simulink model "PlantModel"  (R2022b)
settings: configuration reference "simConfigSet" (kept outside this file)
undefined symbols (not defined in the file): Earth, env, F, GPSTimeSeed, Light, MIL, sensors, uavData, WGS84
libraries: mbdriLib x22, aerolibactuator x5, aerolibasang x2, aerolibatmos2 x2, aerolibconvert2 x2, aerolibwind2 x2, shared6dof x1, aerolibnav x1, simulink x1, aerolibtransform2 x1
(part 1 of 2)
settings Model: Creator=promero  LastModifiedBy=nitinmiyyapuram
settings ConfigSetRef: SourceName=simConfigSet  SourceLocation=Base Workspace

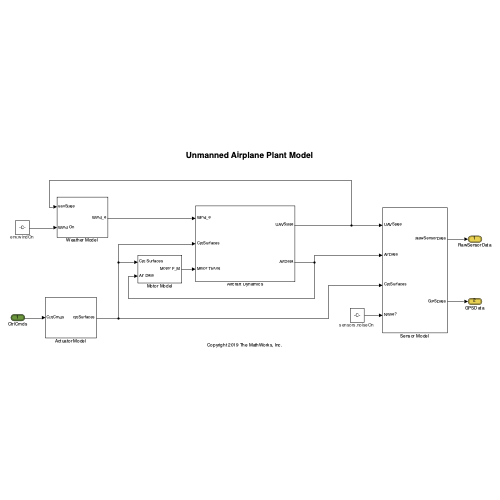
[thumbnail: Simulink's stored preview of the top-level diagram]
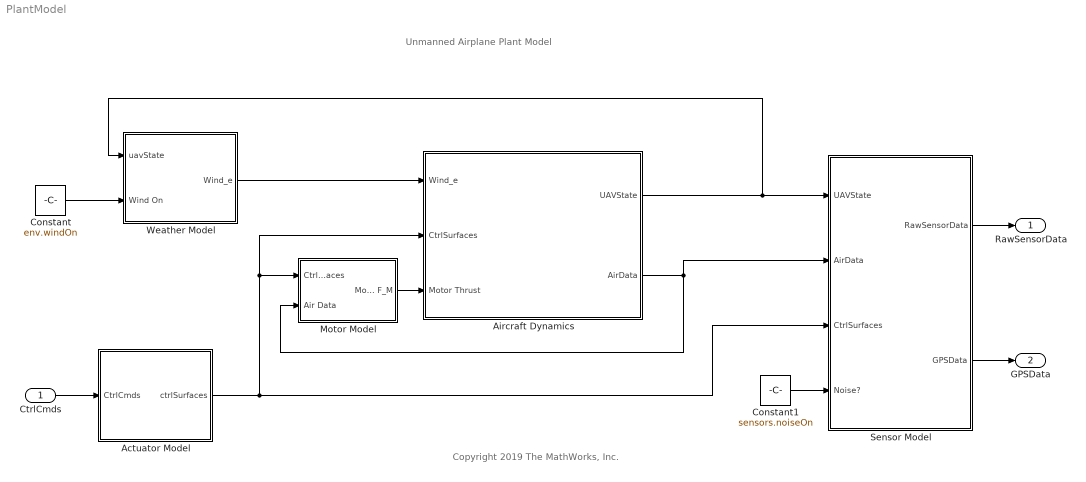
== system PlantModel ==
  note: Unmanned Airplane Plant Model
  note: Copyright 2019 The MathWorks, Inc.
  CtrlCmds : Inport  OutDataTypeStr=Bus: ctrlCmdsBus
  Actuator Model : Subsystem
  Aircraft Dynamics : Subsystem
  Constant : Constant  Value=env.windOn
      settings: AttributesFormatString=%<Value>
  Constant1 : Constant  Value=sensors.noiseOn
      settings: AttributesFormatString=%<Value>
  Motor Model : Subsystem
  Sensor Model : Subsystem
  Weather Model : Subsystem
  RawSensorData : Outport  OutDataTypeStr=Bus: rawSensorDataBus  PortDimensions=1  SampleTime=0  VectorParamsAs1DForOutWhenUnconnected=off  BusOutputAsStruct=on
  GPSData : Outport  Port=2  OutDataTypeStr=Bus: gpsReading  PortDimensions=1  VectorParamsAs1DForOutWhenUnconnected=off  BusOutputAsStruct=on
  wires:
  Sensor Model/2(GPSData) -> GPSData/1
  Weather Model/1(Wind_e) -> Aircraft Dynamics/1(Wind_e)
  Sensor Model/1(RawSensorData) -> RawSensorData/1
  Constant1/1 -> Sensor Model/4(Noise?)
  Constant/1 -> Weather Model/2(Wind On)
  Aircraft Dynamics/1(UAVState) -> Weather Model/1(uavState), Sensor Model/1(UAVState)
  CtrlCmds/1 -> Actuator Model/1(CtrlCmds)
  Actuator Model/1(ctrlSurfaces) -> Sensor Model/3(CtrlSurfaces), Aircraft Dynamics/2(CtrlSurfaces), Motor Model/1(Ctrl Surfaces)
  Motor Model/1(Motor F_M) -> Aircraft Dynamics/3(Motor Thrust)
  Aircraft Dynamics/2(AirData) -> Motor Model/2(Air Data), Sensor Model/2(AirData)

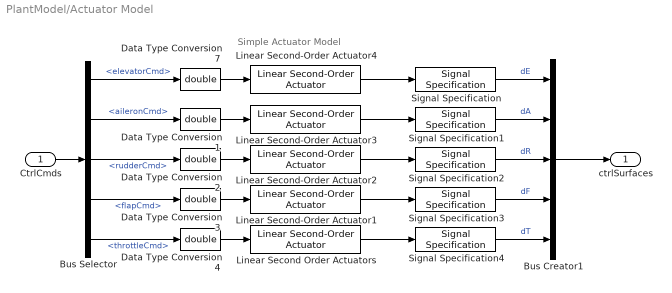
== system PlantModel/Actuator Model ==
  note: Simple Actuator Model
  CtrlCmds : Inport
  Bus Creator1 : BusCreator  Inputs=5
  Bus Selector : BusSelector  OutputSignals=elevatorCmd,aileronCmd,rudderCmd,flapCmd,throttleCmd
  Data Type Conversion{1..4,7} (5 alike) : DataTypeConversion  OutDataTypeStr=double  SaturateOnIntegerOverflow=off  RndMeth=Floor
  Linear Second Order Actuators : aerolibactuator/Linear Second-Order Actuator  wn_fin=35  z_fin=0.75  fin_act_0=0  fin_act_vel=0
      settings: AttributesFormatString=|
      | Nat Freq => %<wn_fin>
      | Damping => %<z_fin>
  Linear Second-Order Actuator{1..4} (4 alike) : aerolibactuator/Linear Second-Order Actuator  wn_fin=35  z_fin=0.75  fin_act_0=0  fin_act_vel=0
  Signal Specification{,1..3} (4 alike) : SignalSpecification  Unit=rad
  Signal Specification4 : SignalSpecification  Unit=%
  ctrlSurfaces : Outport  VectorParamsAs1DForOutWhenUnconnected=off
  wires:
  CtrlCmds/1 -> Bus Selector/1
  Data Type Conversion7/1 -> Linear Second-Order Actuator4/1
  Data Type Conversion1/1 -> Linear Second-Order Actuator3/1
  Data Type Conversion2/1 -> Linear Second-Order Actuator2/1
  Data Type Conversion3/1 -> Linear Second-Order Actuator1/1
  Data Type Conversion4/1 -> Linear Second Order Actuators/1
  Bus Creator1/1 -> ctrlSurfaces/1
  Bus Selector/1 -> Data Type Conversion7/1  "<elevatorCmd>"
  Linear Second-Order Actuator2/1 -> Signal Specification2/1
  Linear Second-Order Actuator3/1 -> Signal Specification1/1
  Linear Second-Order Actuator1/1 -> Signal Specification3/1
  Linear Second-Order Actuator4/1 -> Signal Specification/1
  Bus Selector/4 -> Data Type Conversion3/1  "<flapCmd>"
  Bus Selector/5 -> Data Type Conversion4/1  "<throttleCmd>"
  Bus Selector/3 -> Data Type Conversion2/1  "<rudderCmd>"
  Bus Selector/2 -> Data Type Conversion1/1  "<aileronCmd>"
  Linear Second Order Actuators/1 -> Signal Specification4/1
  Signal Specification/1 -> Bus Creator1/1  "dE"
  Signal Specification1/1 -> Bus Creator1/2  "dA"
  Signal Specification2/1 -> Bus Creator1/3  "dR"
  Signal Specification3/1 -> Bus Creator1/4  "dF"
  Signal Specification4/1 -> Bus Creator1/5  "dT"

== system PlantModel/Aircraft Dynamics ==
  Wind_e : Inport
  CtrlSurfaces : Inport  Port=2
  Motor Thrust : Inport  Port=3
  6DOF Equations of Motion : Subsystem  VariantControl=use_aerospace_blocks == 1
  Aerodynamic Forces and Moments : Subsystem
  Sum : Sum  Inputs=++|  SaturateOnIntegerOverflow=on
  UAVState : Outport  VectorParamsAs1DForOutWhenUnconnected=off
  AirData : Outport  Port=2  VectorParamsAs1DForOutWhenUnconnected=off
  wires:
  Aerodynamic Forces and Moments/1(AirData) -> AirData/1
  6DOF Equations of Motion/1(UAVState) -> UAVState/1, Aerodynamic Forces and Moments/3(UAVState)
  Aerodynamic Forces and Moments/2(FM_b) -> Sum/2
  Sum/1 -> 6DOF Equations of Motion/1(FM_b)
  CtrlSurfaces/1 -> Aerodynamic Forces and Moments/1(CtrlSurfaces)
  Wind_e/1 -> Aerodynamic Forces and Moments/2(Wind_e)
  Motor Thrust/1 -> Sum/1

== system PlantModel/Motor Model ==
  Ctrl Surfaces : Inport
  Air Data : Inport  Port=2
  Bus Selector : BusSelector  OutputSignals=dT
  Bus Selector1 : BusSelector  OutputSignals=airpseed
  Constant : Constant  Value=[0 0 0]
  Engine Model : Subsystem
  Mux : Mux  Inputs=2
  Motor F_M : Outport  VectorParamsAs1DForOutWhenUnconnected=off
  wires:
  Bus Selector1/1 -> Engine Model/2(Airspeed)  "<airpseed>"
  Ctrl Surfaces/1 -> Bus Selector/1
  Engine Model/1(Thrust_b) -> Mux/1
  Constant/1 -> Mux/2
  Air Data/1 -> Bus Selector1/1
  Bus Selector/1 -> Engine Model/1(dt)  "<dT>"
  Mux/1 -> Motor F_M/1

== system PlantModel/Sensor Model ==
  UAVState : Inport
  AirData : Inport  Port=2
  CtrlSurfaces : Inport  Port=3
  Noise? : Inport  Port=4  OutDataTypeStr=double  PortDimensions=1
  "Air Sensor Model " : Subsystem
  Assemble GPS and State Data : Subsystem
  Noise Model : Subsystem  TreatAsAtomicUnit=on
  Sampling Model : Subsystem  TreatAsAtomicUnit=on
  RawSensorData : Outport  OutDataTypeStr=Bus: rawSensorDataBus  PortDimensions=1  SampleTime=0  VectorParamsAs1DForOutWhenUnconnected=off  BusOutputAsStruct=on
  GPSData : Outport  Port=2  OutDataTypeStr=Bus: gpsReading  PortDimensions=1  VectorParamsAs1DForOutWhenUnconnected=off  BusOutputAsStruct=on
  wires:
  Sampling Model/2(GPSData) -> GPSData/1
  Sampling Model/1(RawSensorData) -> RawSensorData/1
  CtrlSurfaces/1 -> Assemble GPS and State Data/3(CtrlSurfaces)
  UAVState/1 -> Assemble GPS and State Data/1(UAVState), "Air Sensor Model "/1(uavState)
  Assemble GPS and State Data/1(UAVStateBus) -> Noise Model/1(UAVState)  "uavState"
  Noise?/1 -> Noise Model/2(Noise?)
  Noise Model/1(SensorData) -> Sampling Model/1(Sensor Data)
  AirData/1 -> "Air Sensor Model "/2(AirData)
  "Air Sensor Model "/1(AirSensorData) -> Assemble GPS and State Data/2(AirSensorData)

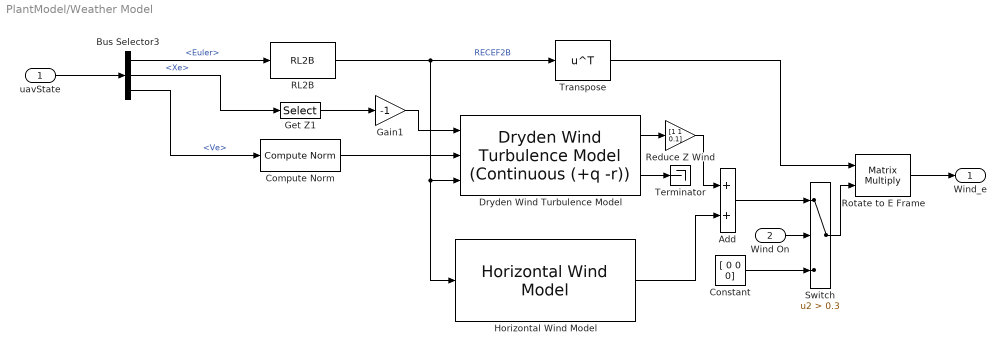
== system PlantModel/Weather Model ==
  uavState : Inport
  Wind On : Inport  Port=2
  " Compute Norm" : mbdriLib/Utilities/ Compute Norm  SystemSampleTime=-1  VariantActivationTime=update diagram  Latency=0  AutoFrameSizeCalculation=off
  Add : Sum  Inputs=2
  Bus Selector3 : BusSelector  OutputSignals=Euler,Xe,Ve
  Constant : Constant  Value=[ 0 0 0]
      settings: AttributesFormatString=%<Value>
  Dryden Wind Turbulence Model : aerolibwind2/Dryden Wind Turbulence Model  (Continuous (+q -r))  units=Metric (MKS)  spec=MIL-F-8785C  model=Continuous Dryden (+q -r)  W20=env.windBase/4  Wdeg=env.windDirTurb  TurbProb=10^-2 - Light  L_high=533.4  Wingspan=uavData.geometry.span  ts=ap.apSampleTime  Seed=[23341 23342 23343 23344]  T_on=on
  Gain1 : Gain  Gain=-1
      settings: AttributesFormatString=Z to Alt
  Get Z1 : Selector  InputPortWidth=3  IndexOptions=Index vector (dialog)  Indices=[3]  OutputSizes=[(-2)]
  "Horizontal Wind Model " : aerolibwind2/Horizontal Wind Model  units=Metric (MKS)  Vw_source=Internal  Vwind=env.windBase  W_source=Internal  Wdeg=env.windDirHor
  RL2B : mbdriLib/Coordinates/RL2B  SystemSampleTime=-1  VariantActivationTime=update diagram  Latency=0  AutoFrameSizeCalculation=off
  Reduce Z Wind : Gain  Gain=[1 1 0.1]
      settings: AttributesFormatString=%<Gain>
  Rotate to E Frame : Product  Multiplication=Matrix(*)
  Switch : Switch  Criteria=u2 > Threshold  Threshold=0.3  SaturateOnIntegerOverflow=off  InputSameDT=off
  Terminator : Terminator
  Transpose : Math  Operator=transpose  SignedPower=on
  Wind_e : Outport  Unit=m/s  VectorParamsAs1DForOutWhenUnconnected=off
  wires:
  Bus Selector3/2 -> Get Z1/1  "<Xe>"
  Bus Selector3/1 -> RL2B/1  "<Euler>"
  Dryden Wind Turbulence Model/2 -> Terminator/1
  Constant/1 -> Switch/3
  Get Z1/1 -> Gain1/1
  Bus Selector3/3 -> " Compute Norm"/1  "<Ve>"
  RL2B/1 -> Dryden Wind Turbulence Model/3, "Horizontal Wind Model "/1, Transpose/1  "RECEF2B"
  Transpose/1 -> Rotate to E Frame/1
  Rotate to E Frame/1 -> Wind_e/1
  Switch/1 -> Rotate to E Frame/2
  Dryden Wind Turbulence Model/1 -> Reduce Z Wind/1
  " Compute Norm"/1 -> Dryden Wind Turbulence Model/2
  uavState/1 -> Bus Selector3/1
  Gain1/1 -> Dryden Wind Turbulence Model/1
  "Horizontal Wind Model "/1 -> Add/2
  Reduce Z Wind/1 -> Add/1
  Add/1 -> Switch/1
  Wind On/1 -> Switch/2

== system PlantModel/Aircraft Dynamics/6DOF Equations of Motion ==
  FM_b : Inport
  6DOF (Euler Angles) : shared6dof/6DOF (Euler Angles)  units=Metric (MKS)  mtype=Fixed  rep=Euler Angles  xme_0=uavData.ic.Pos_0.*[1; 1; -1]  Vm_0=uavData.ic.Vb_0  eul_0=uavData.ic.Euler_0  pm_0=uavData.ic.PQR_0  mass_0=uavData.geometry.mass  mass_e=0.5  mass_f=2.0  inertia=eye(3).*[uavData.inertia.Ixx;uavData.inertia.Iyy; uavData.inertia.Izz]  inertia_e=eye(3)  inertia_f=2*eye(3)  k_quat=1.0  vre_flag=on  abi_flag=off  aMode=aMode  xme_statename=''  Vm_statename=''  eul_statename=''  quat_statename=''  pm_statename=''  mass_statename=''
  Bus Creator : BusCreator  Inputs=7
  Compute psi_dot : Subsystem
  Constant : Constant  Value=[0 0 0]
      settings: AttributesFormatString=%<Value>
  Demux2 : Demux  Outputs=2
  Terminator1 : Terminator
  Three-axis Accelerometer : aerolibnav/Three-axis Accelerometer  units=Metric (MKS)  acc=[0 0 0]  gtype=off  dtype_a=off  w_a=190  z_a=0.707  a_sf_cc=[1 0 0; 0 1 0; 0 0 1]  a_bias=[0 0 0]  a_Ts=0  a_rand=off  a_seeds=[23093 23094 23095]  a_pow=[0.001 0.001 0.001]  a_sat="[-inf  -inf  -inf  inf inf inf]"
  "[0, pi] Wrap Around" : Subsystem
  UAVState : Outport  VectorParamsAs1DForOutWhenUnconnected=off
  wires:
  Three-axis Accelerometer/1 -> Bus Creator/6  "Ab"
  Constant/1 -> Three-axis Accelerometer/4
  "[0, pi] Wrap Around"/1(Wrapped) -> Bus Creator/3  "Euler"
  6DOF (Euler Angles)/8 -> Three-axis Accelerometer/1
  6DOF (Euler Angles)/5 -> Bus Creator/4  "Vb"
  6DOF (Euler Angles)/2 -> Bus Creator/2  "Xe"
  6DOF (Euler Angles)/1 -> Bus Creator/1  "Ve"
  Bus Creator/1 -> UAVState/1
  6DOF (Euler Angles)/7 -> Three-axis Accelerometer/3
  6DOF (Euler Angles)/4 -> Terminator1/1
  6DOF (Euler Angles)/3 -> Compute psi_dot/1(Euler), "[0, pi] Wrap Around"/1(Euler)
  6DOF (Euler Angles)/6 -> Compute psi_dot/2(G), Bus Creator/5, Three-axis Accelerometer/2  "pqr"
  FM_b/1 -> Demux2/1
  Demux2/2 -> 6DOF (Euler Angles)/2
  Demux2/1 -> 6DOF (Euler Angles)/1
  Compute psi_dot/1(psi_dot) -> Bus Creator/7  "psi_dot"

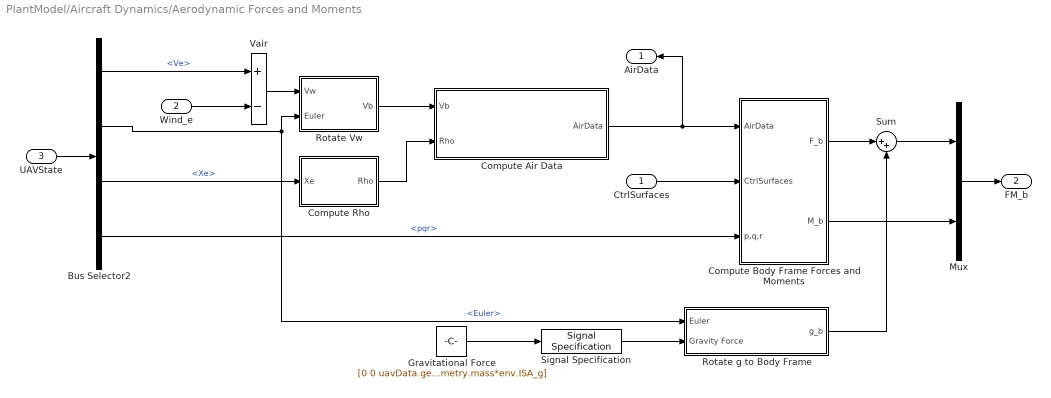
== system PlantModel/Aircraft Dynamics/Aerodynamic Forces and Moments ==
  CtrlSurfaces : Inport
  Wind_e : Inport  Port=2
  UAVState : Inport  Port=3
  Bus Selector2 : BusSelector  OutputSignals=Ve,Euler,Xe,pqr
  Compute Air Data : Subsystem  TreatAsAtomicUnit=on  VariantControl=use_aerospace_blocks == 1
  Compute Body Frame Forces and Moments : Subsystem
  Compute Rho : Subsystem
  Gravitational Force : Constant  Value=[0 0 uavData.geometry.mass*env.ISA_g]  VectorParams1D=off
      settings: AttributesFormatString=%<Value>
  Mux : Mux  Inputs=2
  Rotate Vw : Subsystem
  Rotate g to Body Frame : Subsystem
  Signal Specification : SignalSpecification  Unit=kg*m/s^2
  Sum : Sum  Inputs=|++  SaturateOnIntegerOverflow=on
  Vair : Sum  Inputs=+-  InputSameDT=on  SaturateOnIntegerOverflow=on  OutDataTypeStr=Inherit: Same as first input
  AirData : Outport  VectorParamsAs1DForOutWhenUnconnected=off
  FM_b : Outport  Port=2  VectorParamsAs1DForOutWhenUnconnected=off
  wires:
  Bus Selector2/1 -> Vair/1  "<Ve>"
  UAVState/1 -> Bus Selector2/1
  Mux/1 -> FM_b/1
  Sum/1 -> Mux/1
  Compute Body Frame Forces and Moments/1(F_b) -> Sum/1
  Rotate g to Body Frame/1(g_b) -> Sum/2
  Wind_e/1 -> Vair/2
  CtrlSurfaces/1 -> Compute Body Frame Forces and Moments/2(CtrlSurfaces)
  Compute Air Data/1(AirData) -> AirData/1, Compute Body Frame Forces and Moments/1(AirData)
  Bus Selector2/4 -> Compute Body Frame Forces and Moments/3(p,q,r)  "<pqr>"
  Gravitational Force/1 -> Signal Specification/1
  Compute Body Frame Forces and Moments/2(M_b) -> Mux/2
  Rotate Vw/1(Vb) -> Compute Air Data/1(Vb)
  Compute Rho/1(Rho) -> Compute Air Data/2(Rho)
  Bus Selector2/2 -> Rotate Vw/2(Euler), Rotate g to Body Frame/1(Euler)  "<Euler>"
  Vair/1 -> Rotate Vw/1(Vw)
  Signal Specification/1 -> Rotate g to Body Frame/2(Gravity Force)
  Bus Selector2/3 -> Compute Rho/1(Xe)  "<Xe>"

== system PlantModel/Motor Model/Engine Model ==
  dt : Inport
  Airspeed : Inport  Port=2
  Constant4 : Constant  Value=0
      settings: AttributesFormatString=%<Value>
  Get To : Subsystem
  Mass Conversion : aerolibconvert2/Mass Conversion  IU=lbm  OU=kg
  Mux : Mux  Inputs=2
  Mux1 : Mux  Inputs=3
  Thrust Available (lbs) : Fcn  Expr=u(1) - 0.047*sqrt(u(1))*u(2)
  kg2N : Gain  Gain=env.ISA_g  SaturateOnIntegerOverflow=on  OutDataTypeStr=Inherit: Same as input  ParamDataTypeStr=Inherit: Same as input
      settings: AttributesFormatString=%<Gain>
  Thrust_b : Outport  Unit=kg*m/s^2  VectorParamsAs1DForOutWhenUnconnected=off
  wires:
  kg2N/1 -> Mux1/1
  Constant4/1 -> Mux1/3, Mux1/2
  Mass Conversion/1 -> kg2N/1
  Mux1/1 -> Thrust_b/1
  Airspeed/1 -> Mux/2
  Thrust Available (lbs)/1 -> Mass Conversion/1
  Mux/1 -> Thrust Available (lbs)/1
  Get To/1(To) -> Mux/1
  dt/1 -> Get To/1(dt)

== system PlantModel/Sensor Model/Air Sensor Model  ==
  uavState : Inport
  AirData : Inport  Port=2
  Bus Creator : BusCreator  Inputs=4
  Bus Selector1 : BusSelector  OutputSignals=airpseed,q
  Bus Selector3 : BusSelector  OutputSignals=Xe
  Gain : Gain  Gain=-1
      settings: AttributesFormatString=Z to Alt
  Get Z : Selector  InputPortWidth=3  IndexOptions=Index vector (dialog)  Indices=[3]  OutputSizes=[(-2)]
  ISA Atmosphere Model1 : aerolibatmos2/ISA Atmosphere Model  custom=on  g=env.ISA_g  gamma=1.4  R=env.ISA_R  L=env.ISA_lapse  h_trop=11000  h_strat=20000  rho0=env.ISA_rho0  P0=env.ISA_P0  T0=env.ISA_T0  h0=0
  Terminator : Terminator
  Terminator1 : Terminator
  Transfer Fcn : TransferFcn  Denominator=[.01 1]
  Unit Conversion : UnitConversion  OutputType=Inherit: Inherit via back propagation
  AirSensorData : Outport  VectorParamsAs1DForOutWhenUnconnected=off
  wires:
  Bus Selector3/1 -> Get Z/1  "<Xe>"
  Get Z/1 -> Transfer Fcn/1
  Unit Conversion/1 -> Bus Creator/1  "OAT"
  Bus Selector1/1 -> Bus Creator/3  "<airpseed>"
  Bus Selector1/2 -> Bus Creator/4  "<q>"
  ISA Atmosphere Model1/1 -> Unit Conversion/1  "OAT"
  Bus Creator/1 -> AirSensorData/1
  Gain/1 -> ISA Atmosphere Model1/1
  ISA Atmosphere Model1/3 -> Bus Creator/2  "static"
  ISA Atmosphere Model1/2 -> Terminator1/1
  AirData/1 -> Bus Selector1/1
  Transfer Fcn/1 -> Gain/1
  uavState/1 -> Bus Selector3/1
  ISA Atmosphere Model1/4 -> Terminator/1

== system PlantModel/Sensor Model/Assemble GPS and State Data ==
  UAVState : Inport
  AirSensorData : Inport  Port=2
  CtrlSurfaces : Inport  Port=3
  Bus Creator : BusCreator  Inputs=11  OutDataTypeStr=Bus: uavStateBus  NonVirtualBus=on
      settings: InheritFromInputs=off
  Bus Creator1 : BusCreator  Inputs=5  OutDataTypeStr=Bus: gpsReading
      settings: InheritFromInputs=off
  Bus Selector : BusSelector  OutputSignals=static,q,OAT,airpseed
  Bus Selector1 : BusSelector  OutputSignals=dE,dA,dR,dF,dT
  Bus Selector2 : BusSelector  OutputSignals=Euler,pqr,Xe,Ve,Ab
  Bus Selector3 : BusSelector  OutputSignals=Xe,Ve
  Bus Selector4 : BusSelector  OutputSignals=gps_latLon,gps_h,gps_cog,gps_sog,gps_fix
  Generate GPS Data : Subsystem
  Mux : Mux  Inputs=5
  UAVStateBus : Outport  OutDataTypeStr=Bus: uavStateBus  VectorParamsAs1DForOutWhenUnconnected=off
  wires:
  Bus Creator1/1 -> Bus Creator/10
  Mux/1 -> Bus Creator/11  "ctrlSurfacePos"
  CtrlSurfaces/1 -> Bus Selector1/1  "ctrlSurfacePos"
  Bus Selector1/4 -> Mux/4  "<dF>"
  Bus Selector1/2 -> Mux/2  "<dA>"
  Bus Selector/4 -> Bus Creator/9  "<airpseed>"
  Bus Selector/2 -> Bus Creator/7  "<q>"
  Bus Selector/3 -> Bus Creator/8  "<OAT>"
  Bus Selector1/1 -> Mux/1  "<dE>"
  Bus Selector1/3 -> Mux/3  "<dR>"
  Bus Selector1/5 -> Mux/5  "<dT>"
  Bus Selector/1 -> Bus Creator/6  "<static>"
  Bus Creator/1 -> UAVStateBus/1
  AirSensorData/1 -> Bus Selector/1
  Bus Selector2/5 -> Bus Creator/5  "<Ab>"
  Bus Selector2/1 -> Bus Creator/1  "<Euler>"
  Bus Selector2/3 -> Bus Creator/3  "<Xe>"
  Bus Selector2/4 -> Bus Creator/4  "<Ve>"
  Bus Selector2/2 -> Bus Creator/2  "<pqr>"
  Bus Selector3/1 -> Generate GPS Data/1(XYZ (NEU))  "<Xe>"
  Bus Selector3/2 -> Generate GPS Data/2("Vx, Vy, Vz")  "<Ve>"
  Bus Selector4/5 -> Bus Creator1/5  "<gps_fix>"
  Bus Selector4/1 -> Bus Creator1/1  "<gps_latLon>"
  Bus Selector4/3 -> Bus Creator1/3  "<gps_cog>"
  Generate GPS Data/1(GPSData) -> Bus Selector4/1
  Bus Selector4/4 -> Bus Creator1/4  "<gps_sog>"
  Bus Selector4/2 -> Bus Creator1/2  "<gps_h>"
  UAVState/1 -> Bus Selector3/1, Bus Selector2/1

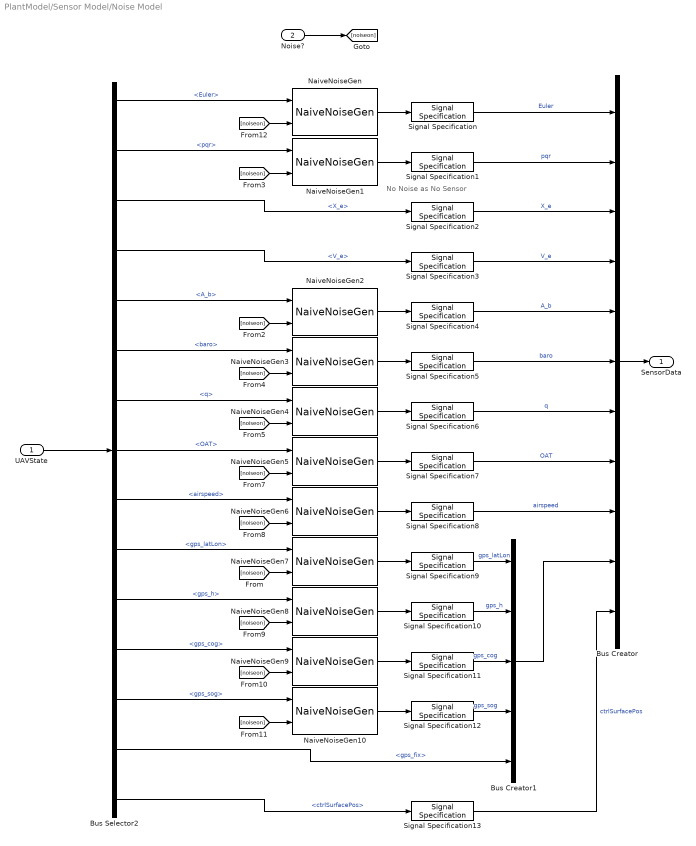
== system PlantModel/Sensor Model/Noise Model ==
  note: No Noise as No Sensor
  UAVState : Inport  OutDataTypeStr=Bus: uavStateBus
  Noise? : Inport  Port=2
  Bus Creator : BusCreator  Inputs=11  OutDataTypeStr=Bus: uavStateBus
      settings: InheritFromInputs=off
  Bus Creator1 : BusCreator  Inputs=5  OutDataTypeStr=Bus: gpsReading
      settings: InheritFromInputs=off
  Bus Selector2 : BusSelector  OutputSignals=Euler,pqr,X_e,V_e,A_b,baro,q,OAT,airspeed,gpsState.gps_latLon,gpsState.gps_h,gpsState.gps_cog,gpsState.gps_sog,gpsState.gps_fix,ctrlSurfacePos
  NaiveNoiseGen : mbdriLib/Utilities/NaiveNoiseGen  np=[0.0005 0.0005 0.0005]  st=ap.apSampleTime  ng=0.05  ns=[132 456 789]
  NaiveNoiseGen1 : mbdriLib/Utilities/NaiveNoiseGen  np=[0.0005 0.0005 0.0005]  st=ap.apSampleTime  ng=0.01  ns=[4132 4456 4789]
  NaiveNoiseGen10 : mbdriLib/Utilities/NaiveNoiseGen  np=[0.0005]  st=ap.apSampleTime  ng=0.1  ns=[8721]
  NaiveNoiseGen2 : mbdriLib/Utilities/NaiveNoiseGen  np=[0.0005 0.0005 0.0005]  st=ap.apSampleTime  ng=0.01  ns=[138 458 788]
  NaiveNoiseGen3 : mbdriLib/Utilities/NaiveNoiseGen  np=[0.0005]  st=ap.apSampleTime  ng=0.2  ns=[1387]
  NaiveNoiseGen4 : mbdriLib/Utilities/NaiveNoiseGen  np=[0.0005]  st=ap.apSampleTime  ng=0.15  ns=[1317]
  NaiveNoiseGen5 : mbdriLib/Utilities/NaiveNoiseGen  np=[0.0005]  st=ap.apSampleTime  ng=0.2  ns=[1917]
  NaiveNoiseGen6 : mbdriLib/Utilities/NaiveNoiseGen  np=[0.0005]  st=ap.apSampleTime  ng=0.15  ns=[1557]
  NaiveNoiseGen7 : mbdriLib/Utilities/NaiveNoiseGen  np=[0.0001 0.0001]  st=ap.apSampleTime  ng=0.00001  ns=[138 458]
  NaiveNoiseGen8 : mbdriLib/Utilities/NaiveNoiseGen  np=[0.0005]  st=ap.apSampleTime  ng=0.15  ns=[7757]
  NaiveNoiseGen9 : mbdriLib/Utilities/NaiveNoiseGen  np=[0.0005]  st=ap.apSampleTime  ng=0.15  ns=[8757]
  Signal Specification : SignalSpecification  Unit=rad
  Signal Specification1 : SignalSpecification  Unit=rad/s
  Signal Specification10 : SignalSpecification  Unit=m
  Signal Specification11 : SignalSpecification  Unit=deg
  Signal Specification12 : SignalSpecification  Unit=m/s
  Signal Specification13 : SignalSpecification  Unit=rad
  Signal Specification2 : SignalSpecification  Unit=m
  Signal Specification3 : SignalSpecification  Unit=m/s
  Signal Specification4 : SignalSpecification  Unit=m/s^2
  Signal Specification5 : SignalSpecification  Unit=Pa
  Signal Specification6 : SignalSpecification  Unit=Pa
  Signal Specification7 : SignalSpecification  Unit=°C
  Signal Specification8 : SignalSpecification  Unit=m/s
  Signal Specification9 : SignalSpecification  Unit=deg
  SensorData : Outport  OutDataTypeStr=Bus: uavStateBus  VectorParamsAs1DForOutWhenUnconnected=off
  wires:
  Bus Selector2/15 -> Signal Specification13/1  "<ctrlSurfacePos>"
  [noiseon] -> NaiveNoiseGen7/2
  Bus Selector2/10 -> NaiveNoiseGen7/1  "<gps_latLon>"
  Bus Selector2/13 -> NaiveNoiseGen10/1  "<gps_sog>"
  [noiseon] -> NaiveNoiseGen10/2
  Bus Selector2/12 -> NaiveNoiseGen9/1  "<gps_cog>"
  [noiseon] -> NaiveNoiseGen9/2
  Bus Selector2/11 -> NaiveNoiseGen8/1  "<gps_h>"
  [noiseon] -> NaiveNoiseGen8/2
  NaiveNoiseGen7/1 -> Signal Specification9/1
  Bus Creator/1 -> SensorData/1
  NaiveNoiseGen10/1 -> Signal Specification12/1
  NaiveNoiseGen9/1 -> Signal Specification11/1
  NaiveNoiseGen8/1 -> Signal Specification10/1
  NaiveNoiseGen6/1 -> Signal Specification8/1
  NaiveNoiseGen5/1 -> Signal Specification7/1
  NaiveNoiseGen4/1 -> Signal Specification6/1
  NaiveNoiseGen3/1 -> Signal Specification5/1
  NaiveNoiseGen2/1 -> Signal Specification4/1
  NaiveNoiseGen1/1 -> Signal Specification1/1
  NaiveNoiseGen/1 -> Signal Specification/1
  Bus Selector2/9 -> NaiveNoiseGen6/1  "<airspeed>"
  Bus Selector2/8 -> NaiveNoiseGen5/1  "<OAT>"
  [noiseon] -> NaiveNoiseGen5/2
  [noiseon] -> NaiveNoiseGen6/2
  Bus Selector2/7 -> NaiveNoiseGen4/1  "<q>"
  Bus Selector2/6 -> NaiveNoiseGen3/1  "<baro>"
  Bus Selector2/5 -> NaiveNoiseGen2/1  "<A_b>"
  Bus Selector2/4 -> Signal Specification3/1  "<V_e>"
  Bus Selector2/3 -> Signal Specification2/1  "<X_e>"
  Bus Selector2/2 -> NaiveNoiseGen1/1  "<pqr>"
  Bus Selector2/1 -> NaiveNoiseGen/1  "<Euler>"
  [noiseon] -> NaiveNoiseGen1/2
  Noise?/1 -> [noiseon]
  [noiseon] -> NaiveNoiseGen3/2
  [noiseon] -> NaiveNoiseGen4/2
  [noiseon] -> NaiveNoiseGen2/2
  [noiseon] -> NaiveNoiseGen/2
  UAVState/1 -> Bus Selector2/1
  Signal Specification/1 -> Bus Creator/1  "Euler"
  Signal Specification1/1 -> Bus Creator/2  "pqr"
  Signal Specification2/1 -> Bus Creator/3  "X_e"
  Signal Specification3/1 -> Bus Creator/4  "V_e"
  Signal Specification4/1 -> Bus Creator/5  "A_b"
  Signal Specification5/1 -> Bus Creator/6  "baro"
  Signal Specification6/1 -> Bus Creator/7  "q"
  Signal Specification7/1 -> Bus Creator/8  "OAT"
  Signal Specification8/1 -> Bus Creator/9  "airspeed"
  Signal Specification13/1 -> Bus Creator/11  "ctrlSurfacePos"
  Signal Specification9/1 -> Bus Creator1/1  "gps_latLon"
  Signal Specification10/1 -> Bus Creator1/2  "gps_h"
  Signal Specification11/1 -> Bus Creator1/3  "gps_cog"
  Signal Specification12/1 -> Bus Creator1/4  "gps_sog"
  Bus Selector2/14 -> Bus Creator1/5  "<gps_fix>"
  Bus Creator1/1 -> Bus Creator/10

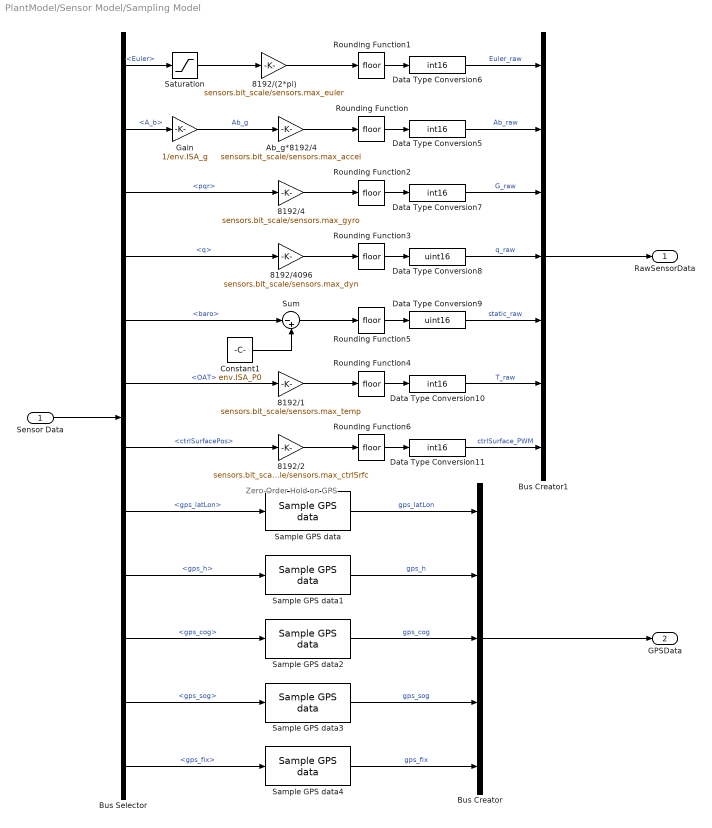
== system PlantModel/Sensor Model/Sampling Model ==
  note: Zero-Order Hold on GPS
  Sensor Data : Inport  OutDataTypeStr=Bus: uavStateBus
  8192/(2*pi) : Gain  Gain=sensors.bit_scale/sensors.max_euler
      settings: AttributesFormatString=%<Gain>
  8192/1 : Gain  Gain=sensors.bit_scale/sensors.max_temp
      settings: AttributesFormatString=%<Gain>
  8192/2 : Gain  Gain=sensors.bit_scale/sensors.max_ctrlSrfc
      settings: AttributesFormatString=%<Gain>
  8192/4 : Gain  Gain=sensors.bit_scale/sensors.max_gyro
      settings: AttributesFormatString=%<Gain>
  8192/4096 : Gain  Gain=sensors.bit_scale/sensors.max_dyn
      settings: AttributesFormatString=%<Gain>
  Ab_g*8192/4 : Gain  Gain=sensors.bit_scale/sensors.max_accel
      settings: AttributesFormatString=%<Gain>
  Bus Creator : BusCreator  Inputs=5  OutDataTypeStr=Bus: gpsReading  NonVirtualBus=on
      settings: InheritFromInputs=off
  Bus Creator1 : BusCreator  Inputs=7  OutDataTypeStr=Bus: rawSensorDataBus  NonVirtualBus=on
  Bus Selector : BusSelector  OutputSignals=Euler,A_b,pqr,q,baro,OAT,ctrlSurfacePos,gpsState.gps_latLon,gpsState.gps_h,gpsState.gps_cog,gpsState.gps_sog,gpsState.gps_fix
  Constant1 : Constant  Value=env.ISA_P0
      settings: AttributesFormatString=%<Value>
  Data Type Conversion{5..7,10..11} (5 alike) : DataTypeConversion  OutDataTypeStr=int16  SaturateOnIntegerOverflow=off  RndMeth=Floor
  Data Type Conversion8 : DataTypeConversion  OutDataTypeStr=uint16  SaturateOnIntegerOverflow=off  RndMeth=Floor
  Data Type Conversion9 : DataTypeConversion  OutDataTypeStr=uint16  SaturateOnIntegerOverflow=off  RndMeth=Floor
  Gain : Gain  Gain=1/env.ISA_g
      settings: AttributesFormatString=%<Gain>
  Rounding Function{,1..6} (7 alike) : Rounding
  Sample GPS data{,1..4} (5 alike) : mbdriLib/Utilities/Sample GPS data  SystemSampleTime=-1  VariantActivationTime=update diagram  Latency=0  AutoFrameSizeCalculation=off
  Saturation : Saturate  UpperLimit=6.28  LowerLimit=-6.28
      settings: AttributesFormatString="[%<LowerLimit>  %<UpperLimit>]"
  Sum : Sum  Inputs=|-+
  RawSensorData : Outport  OutDataTypeStr=Bus: rawSensorDataBus  VectorParamsAs1DForOutWhenUnconnected=off
  GPSData : Outport  Port=2  OutDataTypeStr=Bus: gpsReading  VectorParamsAs1DForOutWhenUnconnected=off
  wires:
  Saturation/1 -> 8192/(2*pi)/1
  Bus Selector/7 -> 8192/2/1  "<ctrlSurfacePos>"
  Data Type Conversion11/1 -> Bus Creator1/7  "ctrlSurface_PWM"
  Rounding Function6/1 -> Data Type Conversion11/1
  8192/2/1 -> Rounding Function6/1
  Bus Creator/1 -> GPSData/1
  Bus Creator1/1 -> RawSensorData/1
  Data Type Conversion6/1 -> Bus Creator1/1  "Euler_raw"
  Data Type Conversion5/1 -> Bus Creator1/2  "Ab_raw"
  Data Type Conversion7/1 -> Bus Creator1/3  "G_raw"
  Data Type Conversion8/1 -> Bus Creator1/4  "q_raw"
  Data Type Conversion9/1 -> Bus Creator1/5  "static_raw"
  Data Type Conversion10/1 -> Bus Creator1/6  "T_raw"
  Rounding Function5/1 -> Data Type Conversion9/1
  Sum/1 -> Rounding Function5/1
  Constant1/1 -> Sum/2
  Rounding Function4/1 -> Data Type Conversion10/1
  8192/1/1 -> Rounding Function4/1
  Rounding Function3/1 -> Data Type Conversion8/1
  8192/4096/1 -> Rounding Function3/1
  Bus Selector/6 -> 8192/1/1  "<OAT>"
  Bus Selector/5 -> Sum/1  "<baro>"
  Bus Selector/4 -> 8192/4096/1  "<q>"
  Bus Selector/3 -> 8192/4/1  "<pqr>"
  8192/4/1 -> Rounding Function2/1
  Rounding Function2/1 -> Data Type Conversion7/1
  8192/(2*pi)/1 -> Rounding Function1/1
  Rounding Function1/1 -> Data Type Conversion6/1
  Rounding Function/1 -> Data Type Conversion5/1
  Ab_g*8192/4/1 -> Rounding Function/1
  Gain/1 -> Ab_g*8192/4/1  "Ab_g"
  Bus Selector/2 -> Gain/1  "<A_b>"
  Bus Selector/8 -> Sample GPS data/1  "<gps_latLon>"
  Bus Selector/9 -> Sample GPS data1/1  "<gps_h>"
  Bus Selector/10 -> Sample GPS data2/1  "<gps_cog>"
  Bus Selector/11 -> Sample GPS data3/1  "<gps_sog>"
  Bus Selector/12 -> Sample GPS data4/1  "<gps_fix>"
  Sample GPS data4/1 -> Bus Creator/5  "gps_fix"
  Sample GPS data3/1 -> Bus Creator/4  "gps_sog"
  Sample GPS data2/1 -> Bus Creator/3  "gps_cog"
  Sample GPS data1/1 -> Bus Creator/2  "gps_h"
  Sample GPS data/1 -> Bus Creator/1  "gps_latLon"
  Sensor Data/1 -> Bus Selector/1
  Bus Selector/1 -> Saturation/1  "<Euler>"

== system PlantModel/Aircraft Dynamics/6DOF Equations of Motion/Compute psi_dot ==
  Euler : Inport
  G : Inport  Port=2
  Mux1 : Mux  Inputs=2
  psidot : Fcn  Expr=(u[5]*sin(u[1])+u[6]*cos(u[1]))/cos(u[2])
  psi_dot : Outport  Unit=rad/S  VectorParamsAs1DForOutWhenUnconnected=off
  wires:
  G/1 -> Mux1/2
  psidot/1 -> psi_dot/1  "psi_dot"
  Mux1/1 -> psidot/1
  Euler/1 -> Mux1/1

== system PlantModel/Aircraft Dynamics/6DOF Equations of Motion/[0, pi] Wrap Around ==
  Euler : Inport
  Compare To Zero : simulink/Logic and Bit Operations/Compare To Zero  relop=>=  OutDataTypeStr=uint8  ZeroCross=off
  Logical Operator : Logic  Operator=NOT  AllPortsSameDT=off  OutDataTypeStr=boolean
  Merge : Merge  InitialOutput=0
  Mux2 : Mux  Inputs=2
  Negative Yaw : Subsystem
  Positive Yaw : Subsystem
  Selector1 : Selector  InputPortWidth=3  IndexOptions=Index vector (dialog)  Indices=[1 2]  OutputSizes=1
  Selector2 : Selector  InputPortWidth=3  IndexOptions=Index vector (dialog)  Indices=[3]  OutputSizes=1
  Wrapped : Outport  VectorParamsAs1DForOutWhenUnconnected=off
  wires:
  Negative Yaw/1(yaw_wr) -> Merge/2
  Positive Yaw/1(yaw_wr) -> Merge/1
  Merge/1 -> Mux2/2
  Logical Operator/1 -> Negative Yaw/Enable
  Compare To Zero/1 -> Logical Operator/1, Positive Yaw/Enable
  Selector2/1 -> Negative Yaw/1(yaw), Positive Yaw/1(yaw), Compare To Zero/1
  Mux2/1 -> Wrapped/1
  Selector1/1 -> Mux2/1
  Euler/1 -> Selector1/1, Selector2/1

== system PlantModel/Aircraft Dynamics/Aerodynamic Forces and Moments/Compute Air Data ==
  Vb : Inport  PortDimensions=3
  Rho : Inport  Port=2
  Bus Creator : BusCreator  Inputs=4
  Dynamic Pressure : aerolibasang/Dynamic Pressure
  "Incidence, Sideslip, & Airspeed" : aerolibasang/Incidence, Sideslip, & Airspeed
  AirData : Outport  VectorParamsAs1DForOutWhenUnconnected=off
  wires:
  Bus Creator/1 -> AirData/1
  "Incidence, Sideslip, & Airspeed"/1 -> Bus Creator/1  "alpha"
  Rho/1 -> Dynamic Pressure/2
  "Incidence, Sideslip, & Airspeed"/3 -> Bus Creator/3  "airpseed"
  Dynamic Pressure/1 -> Bus Creator/4  "q"
  Vb/1 -> "Incidence, Sideslip, & Airspeed"/1, Dynamic Pressure/1
  "Incidence, Sideslip, & Airspeed"/2 -> Bus Creator/2  "beta"

== system PlantModel/Aircraft Dynamics/Aerodynamic Forces and Moments/Compute Body Frame Forces and Moments ==
  AirData : Inport
  CtrlSurfaces : Inport  Port=2
  p,q,r : Inport  Port=3
  Bus Selector : BusSelector  OutputSignals=alpha,beta
  Mux : Mux  Inputs=2
  Rotate FM to body frame : Subsystem
  Wind frame F& M : Subsystem
  F_b : Outport  Unit=kg*m/s^2  VectorParamsAs1DForOutWhenUnconnected=off
  M_b : Outport  Port=2  Unit=kg*m/s  VectorParamsAs1DForOutWhenUnconnected=off
  wires:
  Mux/1 -> Rotate FM to body frame/2(alpha_beta)
  Bus Selector/2 -> Mux/2  "<beta>"
  Bus Selector/1 -> Mux/1  "<alpha>"
  Wind frame F& M/1(FM_w) -> Rotate FM to body frame/1(FM_w)  "FM_W"
  p,q,r/1 -> Wind frame F& M/3(p,q,r)
  Rotate FM to body frame/2(M_b) -> M_b/1
  Rotate FM to body frame/1(F_b) -> F_b/1
  CtrlSurfaces/1 -> Wind frame F& M/2(CtrlSurfaces)
  AirData/1 -> Wind frame F& M/1(Airdata), Bus Selector/1

== system PlantModel/Aircraft Dynamics/Aerodynamic Forces and Moments/Compute Rho ==
  Xe : Inport
  Gain : Gain  Gain=-1
      settings: AttributesFormatString=Z to Alt
  Get Z : Selector  InputPortWidth=3  IndexOptions=Index vector (dialog)  Indices=[3]  OutputSizes=[(-2)]
  ISA Atmosphere Model1 : aerolibatmos2/ISA Atmosphere Model  custom=on  g=env.ISA_g  gamma=1.4  R=env.ISA_R  L=env.ISA_lapse  h_trop=11000  h_strat=20000  rho0=env.ISA_rho0  P0=env.ISA_P0  T0=env.ISA_T0  h0=0
  Terminator : Terminator
  Terminator1 : Terminator
  Terminator2 : Terminator
  Transfer Fcn : TransferFcn  Denominator=[.01 1]
  Rho : Outport  VectorParamsAs1DForOutWhenUnconnected=off
  wires:
  ISA Atmosphere Model1/2 -> Terminator1/1
  ISA Atmosphere Model1/1 -> Terminator/1  "OAT"
  Gain/1 -> ISA Atmosphere Model1/1
  Get Z/1 -> Transfer Fcn/1
  Transfer Fcn/1 -> Gain/1
  ISA Atmosphere Model1/3 -> Terminator2/1  "static"
  Xe/1 -> Get Z/1
  ISA Atmosphere Model1/4 -> Rho/1

== system PlantModel/Aircraft Dynamics/Aerodynamic Forces and Moments/Rotate Vw ==
  Vw : Inport
  Euler : Inport  Port=2
  RL2B : mbdriLib/Coordinates/RL2B  SystemSampleTime=-1  VariantActivationTime=update diagram  Latency=0  AutoFrameSizeCalculation=off
  RL2B * Vw : Product  Multiplication=Matrix(*)  InputSameDT=on  SaturateOnIntegerOverflow=on  OutDataTypeStr=Inherit: Same as first input
  Vb : Outport  Unit=m/s  VectorParamsAs1DForOutWhenUnconnected=off
  wires:
  RL2B * Vw/1 -> Vb/1
  Vw/1 -> RL2B * Vw/2
  RL2B/1 -> RL2B * Vw/1
  Euler/1 -> RL2B/1

== system PlantModel/Aircraft Dynamics/Aerodynamic Forces and Moments/Rotate g to Body Frame ==
  Euler : Inport
  Gravity Force : Inport  Port=2  PortDimensions=3
  Product1 : Product  Multiplication=Matrix(*)  InputSameDT=on  SaturateOnIntegerOverflow=on  OutDataTypeStr=Inherit: Same as first input
  RL2B : mbdriLib/Coordinates/RL2B  SystemSampleTime=-1  VariantActivationTime=update diagram  Latency=0  AutoFrameSizeCalculation=off
  g_b : Outport  Unit=kg*m/s^2  VectorParamsAs1DForOutWhenUnconnected=off
  wires:
  Gravity Force/1 -> Product1/2
  Euler/1 -> RL2B/1
  Product1/1 -> g_b/1
  RL2B/1 -> Product1/1

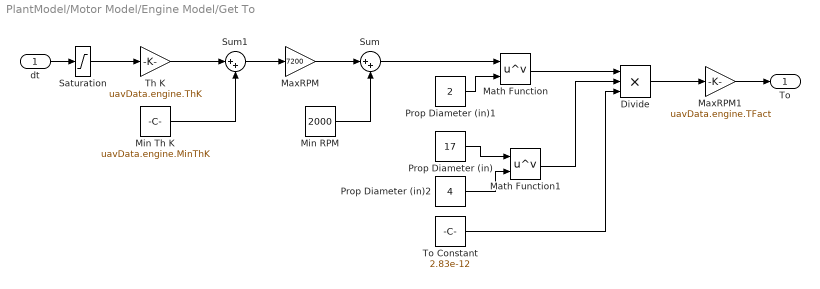
== system PlantModel/Motor Model/Engine Model/Get To ==
  dt : Inport
  Divide : Product  Inputs=3
  Math Function : Math  Operator=pow  SignedPower=on
  Math Function1 : Math  Operator=pow  SignedPower=on
  MaxRPM : Gain  Gain=7200  SaturateOnIntegerOverflow=on  OutDataTypeStr=Inherit: Same as input  ParamDataTypeStr=Inherit: Same as input
      settings: AttributesFormatString=%<Gain>
  MaxRPM1 : Gain  Gain=uavData.engine.TFact  SaturateOnIntegerOverflow=on  OutDataTypeStr=Inherit: Same as input  ParamDataTypeStr=Inherit: Same as input
      settings: AttributesFormatString=%<Gain>
  Min RPM : Constant  Value=2000
      settings: AttributesFormatString=%<Value>
  Min Th K : Constant  Value=uavData.engine.MinThK
      settings: AttributesFormatString=%<Value>
  Prop Diameter (in) : Constant  Value=17
      settings: AttributesFormatString=%<Value>
  Prop Diameter (in)1 : Constant  Value=2
      settings: AttributesFormatString=%<Value>
  Prop Diameter (in)2 : Constant  Value=4
      settings: AttributesFormatString=%<Value>
  Saturation : Saturate  UpperLimit=1.0  LowerLimit=0
      settings: AttributesFormatString="[%<LowerLimit>  %<UpperLimit>]"
  Sum : Sum  Inputs=|++
  Sum1 : Sum  Inputs=|++
  Th K : Gain  Gain=uavData.engine.ThK  SaturateOnIntegerOverflow=on  OutDataTypeStr=Inherit: Same as input  ParamDataTypeStr=Inherit: Same as input
      settings: AttributesFormatString=%<Gain>
  To Constant : Constant  Value=2.83e-12
      settings: AttributesFormatString=%<Value>
  To : Outport  VectorParamsAs1DForOutWhenUnconnected=off
  wires:
  Min Th K/1 -> Sum1/2
  Sum1/1 -> MaxRPM/1
  dt/1 -> Saturation/1
  Th K/1 -> Sum1/1
  MaxRPM/1 -> Sum/1
  Min RPM/1 -> Sum/2
  Sum/1 -> Math Function/1
  MaxRPM1/1 -> To/1
  Divide/1 -> MaxRPM1/1
  To Constant/1 -> Divide/3
  Math Function1/1 -> Divide/2
  Math Function/1 -> Divide/1
  Prop Diameter (in)/1 -> Math Function1/1
  Prop Diameter (in)2/1 -> Math Function1/2
  Prop Diameter (in)1/1 -> Math Function/2
  Saturation/1 -> Th K/1

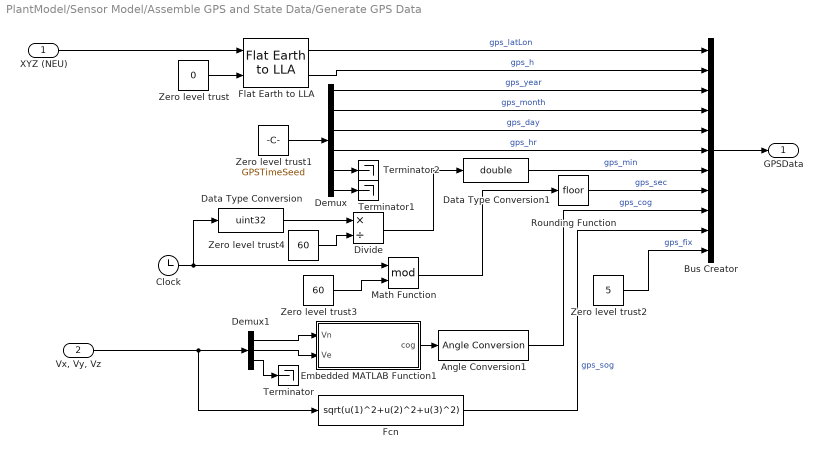
== system PlantModel/Sensor Model/Assemble GPS and State Data/Generate GPS Data ==
  XYZ (NEU) : Inport
  "Vx, Vy, Vz" : Inport  Port=2
  Angle Conversion1 : aerolibconvert2/Angle Conversion  IU=rad  OU=deg
  Bus Creator : BusCreator  Inputs=11
  Clock : Clock
      settings: AttributesFormatString=Decimation: %<Decimation>  Decimation=100
  Data Type Conversion : DataTypeConversion  OutDataTypeStr=uint32  SaturateOnIntegerOverflow=off  RndMeth=Floor
  Data Type Conversion1 : DataTypeConversion  OutDataTypeStr=double  SaturateOnIntegerOverflow=off  RndMeth=Floor
  Demux : Demux  Outputs=6
  Demux1 : Demux  Outputs=3
  Divide : Product  Inputs=*/  OutDataTypeStr=uint32
  Embedded MATLAB Function1 : MATLAB Function  TreatAsAtomicUnit=on
  Fcn : Fcn  Expr=sqrt(u(1)^2+u(2)^2+u(3)^2)
  Flat Earth to LLA : aerolibtransform2/Flat Earth to LLA  units=Metric (MKS)  ptype=Earth (WGS84)  F=1/298.257223563  R=6378137  refPosPort=off  LL0=uavData.ic.gsLL  psi=0
  Math Function : Math  Operator=mod  SignedPower=on
  Rounding Function : Rounding
  Terminator : Terminator
  Terminator1 : Terminator
  Terminator2 : Terminator
  Zero level trust : Constant  Value=0
      settings: AttributesFormatString=%<Value>
  Zero level trust1 : Constant  Value=GPSTimeSeed  SampleTime=Inf
      settings: AttributesFormatString=%<Value>
  Zero level trust2 : Constant  Value=5  OutDataTypeStr=uint8
      settings: AttributesFormatString=%<Value>
  Zero level trust3 : Constant  Value=60
      settings: AttributesFormatString=%<Value>
  Zero level trust4 : Constant  Value=60  OutDataTypeStr=uint32
      settings: AttributesFormatString=%<Value>
  GPSData : Outport  VectorParamsAs1DForOutWhenUnconnected=off
  wires:
  Zero level trust2/1 -> Bus Creator/11  "gps_fix"
  Bus Creator/1 -> GPSData/1
  Demux/2 -> Bus Creator/4  "gps_month"
  Demux1/3 -> Terminator/1
  Demux/1 -> Bus Creator/3  "gps_year"
  Angle Conversion1/1 -> Bus Creator/9  "gps_cog"
  Embedded MATLAB Function1/1(cog) -> Angle Conversion1/1
  "Vx, Vy, Vz"/1 -> Demux1/1, Fcn/1
  Demux1/2 -> Embedded MATLAB Function1/2(Ve)
  Demux1/1 -> Embedded MATLAB Function1/1(Vn)
  Fcn/1 -> Bus Creator/10  "gps_sog"
  Rounding Function/1 -> Bus Creator/8  "gps_sec"
  Demux/4 -> Bus Creator/6  "gps_hr"
  Demux/3 -> Bus Creator/5  "gps_day"
  Zero level trust1/1 -> Demux/1
  Flat Earth to LLA/1 -> Bus Creator/1  "gps_latLon"
  Zero level trust/1 -> Flat Earth to LLA/2
  XYZ (NEU)/1 -> Flat Earth to LLA/1
  Zero level trust3/1 -> Math Function/2
  Clock/1 -> Data Type Conversion/1, Math Function/1
  Math Function/1 -> Rounding Function/1
  Demux/6 -> Terminator1/1
  Data Type Conversion/1 -> Divide/1
  Zero level trust4/1 -> Divide/2
  Divide/1 -> Data Type Conversion1/1
  Data Type Conversion1/1 -> Bus Creator/7  "gps_min"
  Demux/5 -> Terminator2/1
  Flat Earth to LLA/2 -> Bus Creator/2  "gps_h"

== system PlantModel/Aircraft Dynamics/6DOF Equations of Motion/[0, pi] Wrap Around/Negative Yaw ==
  yaw : Inport
  Enable : EnablePort
  Abs : Abs  SaturateOnIntegerOverflow=off
  Constant1 : Constant  Value=2*pi
      settings: AttributesFormatString=%<Value>
  Constant2 : Constant  Value=2*pi
      settings: AttributesFormatString=%<Value>
  Math Function : Math  Operator=mod  SignedPower=on
  Sum : Sum  Inputs=|-+
  yaw_wr : Outport  VectorParamsAs1DForOutWhenUnconnected=off
  wires:
  Sum/1 -> yaw_wr/1
  Constant2/1 -> Sum/2
  Abs/1 -> Math Function/1
  Math Function/1 -> Sum/1
  Constant1/1 -> Math Function/2
  yaw/1 -> Abs/1

== system PlantModel/Aircraft Dynamics/6DOF Equations of Motion/[0, pi] Wrap Around/Positive Yaw ==
  yaw : Inport
  Enable : EnablePort
  Constant1 : Constant  Value=2*pi
      settings: AttributesFormatString=%<Value>
  Math Function : Math  Operator=mod  SignedPower=on
  yaw_wr : Outport  VectorParamsAs1DForOutWhenUnconnected=off
  wires:
  Math Function/1 -> yaw_wr/1
  Constant1/1 -> Math Function/2
  yaw/1 -> Math Function/1

== system PlantModel/Aircraft Dynamics/Aerodynamic Forces and Moments/Compute Body Frame Forces and Moments/Rotate FM to body frame ==
  FM_w : Inport
  alpha_beta : Inport  Port=2
  Forces : Selector  InputPortWidth=6  IndexOptions=Index vector (dialog)  Indices=[1 2 3]  OutputSizes=[(-2)]
  Moments : Selector  InputPortWidth=6  IndexOptions=Index vector (dialog)  Indices=[4 5 6]  OutputSizes=[(-2)]
  Rotate Forces : Subsystem
  Rotate Moments : Subsystem
  F_b : Outport  VectorParamsAs1DForOutWhenUnconnected=off
  M_b : Outport  Port=2  VectorParamsAs1DForOutWhenUnconnected=off
  wires:
  alpha_beta/1 -> Rotate Forces/2(alpha_beta), Rotate Moments/1(alpha_beta)
  Moments/1 -> Rotate Moments/2(M_w)
  FM_w/1 -> Moments/1, Forces/1
  Forces/1 -> Rotate Forces/1(F_w)
  Rotate Moments/1(M_b) -> M_b/1
  Rotate Forces/1(F_b) -> F_b/1

== system PlantModel/Aircraft Dynamics/Aerodynamic Forces and Moments/Compute Body Frame Forces and Moments/Wind frame F& M ==
  Airdata : Inport
  CtrlSurfaces : Inport  Port=2
  p,q,r : Inport  Port=3
  Bus Creator1 : BusCreator  Inputs=2
  Bus Selector1 : BusSelector  OutputSignals=dA,dR
  Bus Selector2 : BusSelector  OutputSignals=dE,dF
  Bus Selector6 : BusSelector  OutputSignals=beta,airpseed
  Bus Selector7 : BusSelector  OutputSignals=alpha,airpseed
  Get Forces and Moments : Subsystem
  Lateral Channel : Subsystem
  Longitudinal Channel : Subsystem
  FM_w : Outport  PortDimensions=6  VectorParamsAs1DForOutWhenUnconnected=off
  wires:
  Get Forces and Moments/1(FM_w) -> FM_w/1
  Bus Creator1/1 -> Get Forces and Moments/2(AeroCoeffs)
  Bus Selector7/2 -> Longitudinal Channel/2(Airpseed)  "<airpseed>"
  Bus Selector7/1 -> Longitudinal Channel/1(alpha)  "<alpha>"
  Bus Selector6/2 -> Lateral Channel/2(Airspeed)  "<airpseed>"
  Bus Selector6/1 -> Lateral Channel/1(beta)  "<beta>"
  Airdata/1 -> Bus Selector6/1, Bus Selector7/1, Get Forces and Moments/1(Airdata)
  Bus Selector2/2 -> Longitudinal Channel/4(dF)  "<dF>"
  Bus Selector2/1 -> Longitudinal Channel/3(dE)  "<dE>"
  Bus Selector1/2 -> Lateral Channel/4(dR)  "<dR>"
  Bus Selector1/1 -> Lateral Channel/3(dA)  "<dA>"
  CtrlSurfaces/1 -> Bus Selector1/1, Bus Selector2/1
  p,q,r/1 -> Lateral Channel/5(p,q,r), Longitudinal Channel/5(p,q,r)
  Lateral Channel/1(Lateral) -> Bus Creator1/1
  Longitudinal Channel/1(Longitudinal) -> Bus Creator1/2

== system PlantModel/Aircraft Dynamics/Aerodynamic Forces and Moments/Compute Body Frame Forces and Moments/Rotate FM to body frame/Rotate Forces ==
  F_w : Inport
  alpha_beta : Inport  Port=2
  Product2 : Product  Multiplication=Matrix(*)  SaturateOnIntegerOverflow=on  OutDataTypeStr=Inherit: Same as first input
  RB2W : Subsystem
  RW2B : Math  Operator=transpose  SignedPower=on
  F_b : Outport  PortDimensions=3  VectorParamsAs1DForOutWhenUnconnected=off
  wires:
  RW2B/1 -> Product2/1
  F_w/1 -> Product2/2
  Product2/1 -> F_b/1
  alpha_beta/1 -> RB2W/1(aoa beta)
  RB2W/1(Rw2b) -> RW2B/1

== system PlantModel/Aircraft Dynamics/Aerodynamic Forces and Moments/Compute Body Frame Forces and Moments/Rotate FM to body frame/Rotate Moments ==
  alpha_beta : Inport
  M_w : Inport  Port=2
  Product2 : Product  Multiplication=Matrix(*)  SaturateOnIntegerOverflow=on  OutDataTypeStr=Inherit: Same as first input
  RB2W : Subsystem
  RW2B : Math  Operator=transpose  SignedPower=on
  M_b : Outport  PortDimensions=3  VectorParamsAs1DForOutWhenUnconnected=off
  wires:
  RW2B/1 -> Product2/1
  RB2W/1(Rw2b) -> RW2B/1
  alpha_beta/1 -> RB2W/1(aoa beta)
  Product2/1 -> M_b/1
  M_w/1 -> Product2/2

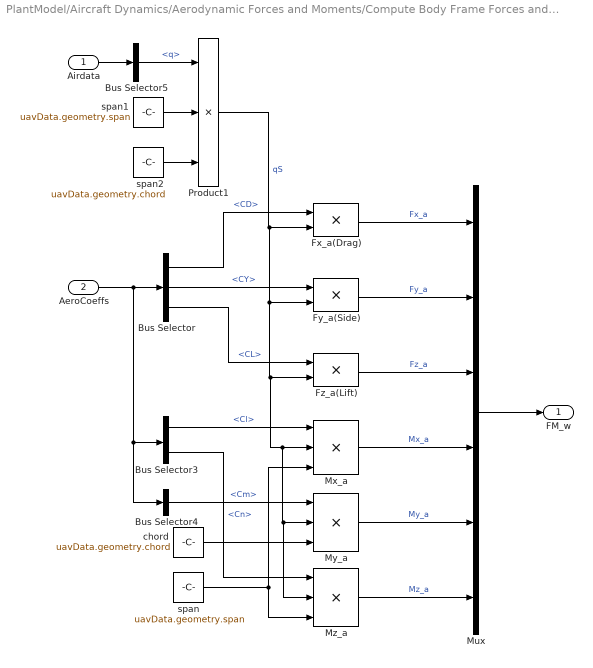
== system PlantModel/Aircraft Dynamics/Aerodynamic Forces and Moments/Compute Body Frame Forces and Moments/Wind frame F& M/Get Forces and Moments ==
  Airdata : Inport
  AeroCoeffs : Inport  Port=2
  Bus Selector : BusSelector  OutputSignals=signal2.CD,signal1.CY,signal2.CL
  Bus Selector3 : BusSelector  OutputSignals=signal1.Cl,signal1.Cn
  Bus Selector4 : BusSelector  OutputSignals=signal2.Cm
  Bus Selector5 : BusSelector  OutputSignals=q
  Fx_a(Drag) : Product  Inputs=**  SaturateOnIntegerOverflow=on  OutDataTypeStr=Inherit: Same as first input
  Fy_a(Side) : Product  SaturateOnIntegerOverflow=on  OutDataTypeStr=Inherit: Same as first input
  Fz_a(Lift) : Product  SaturateOnIntegerOverflow=on  OutDataTypeStr=Inherit: Same as first input
  Mux : Mux  Inputs=6
  Mx_a : Product  Inputs=3  SaturateOnIntegerOverflow=on  OutDataTypeStr=Inherit: Same as first input
  My_a : Product  Inputs=3  SaturateOnIntegerOverflow=on  OutDataTypeStr=Inherit: Same as first input
  Mz_a : Product  Inputs=3  SaturateOnIntegerOverflow=on  OutDataTypeStr=Inherit: Same as first input
  Product1 : Product  Inputs=3  SaturateOnIntegerOverflow=on  OutDataTypeStr=Inherit: Same as first input
  chord : Constant  Value=uavData.geometry.chord  VectorParams1D=off
      settings: AttributesFormatString=%<Value>
  span : Constant  Value=uavData.geometry.span  VectorParams1D=off
      settings: AttributesFormatString=%<Value>
  span1 : Constant  Value=uavData.geometry.span  VectorParams1D=off
      settings: AttributesFormatString=%<Value>
  span2 : Constant  Value=uavData.geometry.chord  VectorParams1D=off
      settings: AttributesFormatString=%<Value>
  FM_w : Outport  VectorParamsAs1DForOutWhenUnconnected=off
  wires:
  Mx_a/1 -> Mux/4  "Mx_a"
  Bus Selector/2 -> Fy_a(Side)/1  "<CY>"
  Bus Selector4/1 -> My_a/1  "<Cm>"
  span2/1 -> Product1/3
  Fx_a(Drag)/1 -> Mux/1  "Fx_a"
  Bus Selector/1 -> Fx_a(Drag)/1  "<CD>"
  AeroCoeffs/1 -> Bus Selector/1, Bus Selector4/1, Bus Selector3/1
  My_a/1 -> Mux/5  "My_a"
  Fz_a(Lift)/1 -> Mux/3  "Fz_a"
  Mz_a/1 -> Mux/6  "Mz_a"
  Airdata/1 -> Bus Selector5/1
  chord/1 -> My_a/3
  span/1 -> Mz_a/3, Mx_a/3
  Fy_a(Side)/1 -> Mux/2  "Fy_a"
  Mux/1 -> FM_w/1
  Bus Selector3/2 -> Mz_a/1  "<Cn>"
  Bus Selector/3 -> Fz_a(Lift)/1  "<CL>"
  Product1/1 -> Fx_a(Drag)/2, Fy_a(Side)/2, Fz_a(Lift)/2, Mx_a/2, My_a/2, Mz_a/2  "qS"
  span1/1 -> Product1/2
  Bus Selector3/1 -> Mx_a/1  "<Cl>"
  Bus Selector5/1 -> Product1/1  "<q>"

== system PlantModel/Aircraft Dynamics/Aerodynamic Forces and Moments/Compute Body Frame Forces and Moments/Wind frame F& M/Lateral Channel ==
  beta : Inport
  Airspeed : Inport  Port=2
  dA : Inport  Port=3
  dR : Inport  Port=4
  p,q,r : Inport  Port=5
  Bus Creator : BusCreator  Inputs=3
  CY : Subsystem
  Cl : Subsystem
  Cn : Subsystem
  Lateral : Outport  VectorParamsAs1DForOutWhenUnconnected=off
  wires:
  Cl/1(Cl) -> Bus Creator/2  "Cl"
  p,q,r/1 -> Cn/4(p,q,r), Cl/4(p,q,r)
  Airspeed/1 -> Cn/5(Airspeed), Cl/5(Airspeed)
  dR/1 -> CY/2(dR), Cl/3(dR), Cn/3(Dr)
  dA/1 -> Cl/2(dA), Cn/2(dA)
  beta/1 -> CY/1(beta), Cl/1(beta), Cn/1(beta)
  Cn/1(Cn) -> Bus Creator/3  "Cn"
  CY/1(CY) -> Bus Creator/1  "CY"
  Bus Creator/1 -> Lateral/1

== system PlantModel/Aircraft Dynamics/Aerodynamic Forces and Moments/Compute Body Frame Forces and Moments/Wind frame F& M/Longitudinal Channel ==
  alpha : Inport
  Airpseed : Inport  Port=2
  dE : Inport  Port=3
  dF : Inport  Port=4
  p,q,r : Inport  Port=5
  Bus Creator : BusCreator  Inputs=3
  CD : Subsystem
  CL : Subsystem
  Cm : Subsystem
  Transfer Fcn : TransferFcn  Numerator=[1 0]  Denominator=[0.1 1]
  Y-down : Gain  Gain=-1  SaturateOnIntegerOverflow=on  OutDataTypeStr=Inherit: Same as input  ParamDataTypeStr=Inherit: Same as input
      settings: AttributesFormatString=%<Gain>
  Longitudinal : Outport  VectorParamsAs1DForOutWhenUnconnected=off
  wires:
  Transfer Fcn/1 -> CL/2(alpha_dot)
  Airpseed/1 -> CL/6(Airspeed)
  p,q,r/1 -> Cm/4(p,q,r), CL/5(p,q,r)
  dF/1 -> Cm/3(Df), CL/4(dF)
  Bus Creator/1 -> Longitudinal/1
  Cm/1(Cm) -> Bus Creator/3  "Cm"
  CL/1(CL) -> CD/1(CL), Y-down/1
  dE/1 -> Cm/2(De), CL/3(dE)
  Y-down/1 -> Bus Creator/2  "CL"
  CD/1(CD) -> Bus Creator/1  "CD"
  alpha/1 -> Transfer Fcn/1, Cm/1(alpha), CL/1(alpha)

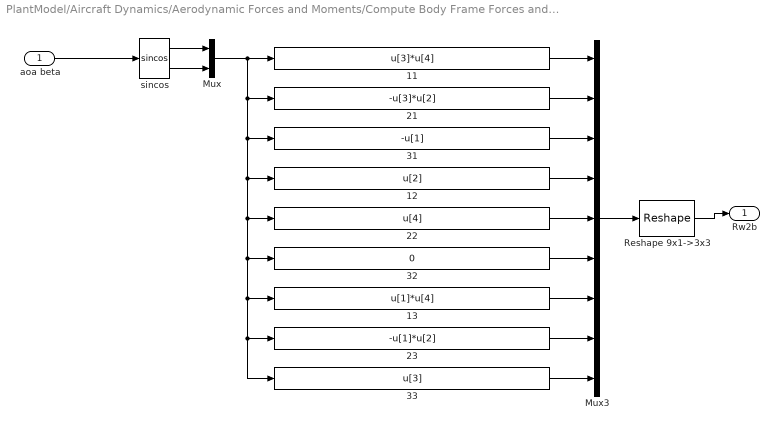
== system PlantModel/Aircraft Dynamics/Aerodynamic Forces and Moments/Compute Body Frame Forces and Moments/Rotate FM to body frame/Rotate Forces/RB2W ==
  aoa beta : Inport
  11 : Fcn  Expr=u[3]*u[4]
  12 : Fcn  Expr=u[2]
  13 : Fcn  Expr=u[1]*u[4]
  21 : Fcn  Expr=-u[3]*u[2]
  22 : Fcn  Expr=u[4]
  23 : Fcn  Expr=-u[1]*u[2]
  31 : Fcn  Expr=-u[1]
  32 : Fcn  Expr=0
  33 : Fcn  Expr=u[3]
  Mux : Mux  Inputs=2
  Mux3 : Mux  Inputs=9
  Reshape 9x1->3x3 : Reshape  OutputDimensionality=Customize  OutputDimensions=[3,3]
  sincos : Trigonometry  Operator=sincos
  Rw2b : Outport  VectorParamsAs1DForOutWhenUnconnected=off
  wires:
  Mux/1 -> 11/1, 21/1, 31/1, 12/1, 22/1, 32/1, 13/1, 23/1, 33/1
  aoa beta/1 -> sincos/1
  sincos/2 -> Mux/2
  sincos/1 -> Mux/1
  33/1 -> Mux3/9
  23/1 -> Mux3/8
  13/1 -> Mux3/7
  32/1 -> Mux3/6
  22/1 -> Mux3/5
  12/1 -> Mux3/4
  31/1 -> Mux3/3
  21/1 -> Mux3/2
  11/1 -> Mux3/1
  Reshape 9x1->3x3/1 -> Rw2b/1
  Mux3/1 -> Reshape 9x1->3x3/1

== system PlantModel/Aircraft Dynamics/Aerodynamic Forces and Moments/Compute Body Frame Forces and Moments/Rotate FM to body frame/Rotate Moments/RB2W ==
  aoa beta : Inport
  11 : Fcn  Expr=u[3]*u[4]
  12 : Fcn  Expr=u[2]
  13 : Fcn  Expr=u[1]*u[4]
  21 : Fcn  Expr=-u[3]*u[2]
  22 : Fcn  Expr=u[4]
  23 : Fcn  Expr=-u[1]*u[2]
  31 : Fcn  Expr=-u[1]
  32 : Fcn  Expr=0
  33 : Fcn  Expr=u[3]
  Mux : Mux  Inputs=2
  Mux3 : Mux  Inputs=9
  Reshape 9x1->3x3 : Reshape  OutputDimensionality=Customize  OutputDimensions=[3,3]
  sincos : Trigonometry  Operator=sincos
  Rw2b : Outport  VectorParamsAs1DForOutWhenUnconnected=off
  wires:
  Mux/1 -> 11/1, 21/1, 31/1, 12/1, 22/1, 32/1, 13/1, 23/1, 33/1
  aoa beta/1 -> sincos/1
  sincos/2 -> Mux/2
  sincos/1 -> Mux/1
  33/1 -> Mux3/9
  23/1 -> Mux3/8
  13/1 -> Mux3/7
  32/1 -> Mux3/6
  22/1 -> Mux3/5
  12/1 -> Mux3/4
  31/1 -> Mux3/3
  21/1 -> Mux3/2
  11/1 -> Mux3/1
  Reshape 9x1->3x3/1 -> Rw2b/1
  Mux3/1 -> Reshape 9x1->3x3/1

== system PlantModel/Aircraft Dynamics/Aerodynamic Forces and Moments/Compute Body Frame Forces and Moments/Wind frame F& M/Lateral Channel/CY ==
  beta : Inport
  dR : Inport  Port=2
  CYDr : Constant  Value=uavData.aero.CYDr
      settings: AttributesFormatString=%<Value>
  CYb : Constant  Value=uavData.aero.CYb
      settings: AttributesFormatString=%<Value>
  Product : Product  SaturateOnIntegerOverflow=on  OutDataTypeStr=Inherit: Same as first input
  Product1 : Product  SaturateOnIntegerOverflow=on  OutDataTypeStr=Inherit: Same as first input
  Sum2 : Sum  SaturateOnIntegerOverflow=on
  CY : Outport  VectorParamsAs1DForOutWhenUnconnected=off
  wires:
  Product1/1 -> Sum2/2
  dR/1 -> Product1/2
  CYDr/1 -> Product1/1
  Product/1 -> Sum2/1
  Sum2/1 -> CY/1
  beta/1 -> Product/2
  CYb/1 -> Product/1
